simulink model "LogisticsMissionPlanEval"  (R2026a)
settings: Solver=VariableStepAuto  StopTime=CAMPAIGN_HR
undefined symbols (not defined in the file or in its folder): DISPATCH_PERIOD_HR, DORMANT_FACTOR, FOB_CONSUMPTION_TPH, FOB_STOCK_INITIAL_TONS, LOSS_FRAC_MAX, LOSS_FRAC_MIN, m, n, P_AMBUSH_NORTH, P_AMBUSH_SOUTH, P_CATASTROPHIC_KILL, RUN_SEED_NORTH, RUN_SEED_SOUTH, SURGE_FACTOR, T_ACTIVE_NORTH_HR, T_ACTIVE_SOUTH_HR, T_DORMANT_NORTH_HR, T_DORMANT_SOUTH_HR, T_SURGE_NORTH_HR, T_SURGE_SOUTH_HR
settings Model: Creator=sarah  LastModifiedBy=sdagen

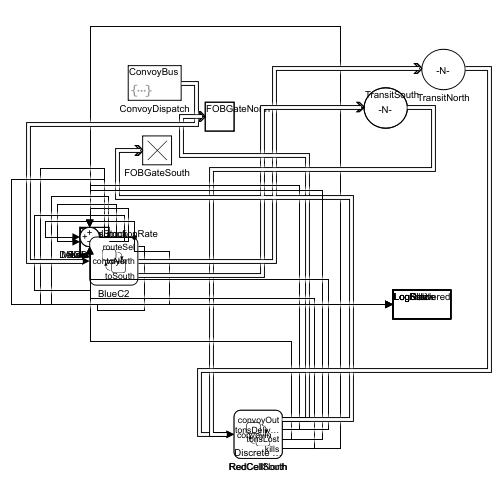
[thumbnail: Simulink's stored preview of the top-level diagram]
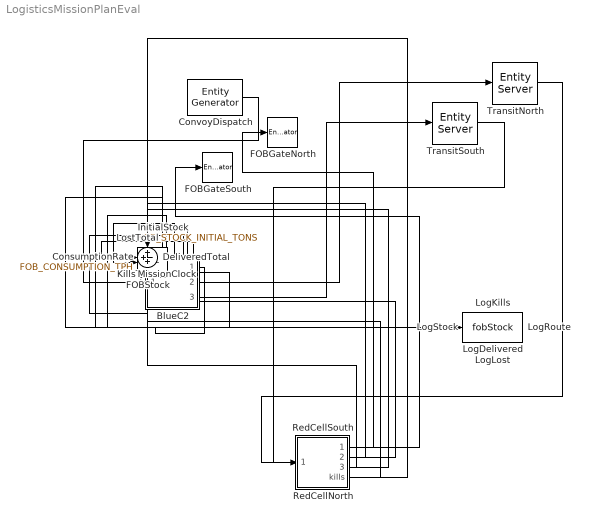
== system LogisticsMissionPlanEval ==
  BlueC2 : Stateflow chart  TreatAsAtomicUnit=on
  ConsumptionRate : Gain  Gain=FOB_CONSUMPTION_TPH
  ConvoyDispatch : EntityGenerator  OutputPortMessageModes=m  Period=DISPATCH_PERIOD_HR  GenerateAction=|  EntityType=Bus object  EntityTypeName=ConvoyBus  DataInitialValue=CONVOY_INIT
      | entity.Trucks = TRUCKS_PER_CONVOY;
      | entity.CargoTons = CONVOY_CARGO_TONS;
  DeliveredTotal : Sum
  FOBGateNorth : EntityTerminator  InputPortMessageModes=m
  FOBGateSouth : EntityTerminator  InputPortMessageModes=m
  FOBStock : Sum  Inputs=++-
  InitialStock : Constant  Value=FOB_STOCK_INITIAL_TONS
  KillsTotal : Sum
  LogDelivered : ToWorkspace  VariableName=deliveredTons  SaveFormat=Timeseries  SampleTime=-1
  LogKills : ToWorkspace  VariableName=convoysKilled  SaveFormat=Timeseries  SampleTime=-1
  LogLost : ToWorkspace  VariableName=lostTons  SaveFormat=Timeseries  SampleTime=-1
  LogRoute : ToWorkspace  VariableName=routeSelected  SaveFormat=Timeseries  SampleTime=-1
  LogStock : ToWorkspace  VariableName=fobStock  SaveFormat=Timeseries  SampleTime=-1
  LostTotal : Sum
  MissionClock : Clock
  RedCellNorth : Stateflow chart  TreatAsAtomicUnit=on
  RedCellSouth : Stateflow chart  TreatAsAtomicUnit=on
  TransitNorth : EntityServer  InputPortMessageModes=m  OutputPortMessageModes=m  Capacity=MAX_CONVOYS_EN_ROUTE  ServiceTimeValue=TRANSIT_NORTH_HR
  TransitSouth : EntityServer  InputPortMessageModes=m  OutputPortMessageModes=m  Capacity=MAX_CONVOYS_EN_ROUTE  ServiceTimeValue=TRANSIT_SOUTH_HR
  wires:
  MissionClock/1 -> ConsumptionRate/1
  InitialStock/1 -> FOBStock/1
  DeliveredTotal/1 -> LogDelivered/1, FOBStock/2
  ConsumptionRate/1 -> FOBStock/3
  LostTotal/1 -> LogLost/1
  KillsTotal/1 -> LogKills/1
  FOBStock/1 -> LogStock/1
  TransitNorth/1 -> RedCellNorth/1(convoyIn)
  TransitSouth/1 -> RedCellSouth/1(convoyIn)
  RedCellNorth/1(convoyOut) -> FOBGateNorth/1
  RedCellSouth/1(convoyOut) -> FOBGateSouth/1
  RedCellNorth/2(tonsDelivered) -> DeliveredTotal/1
  RedCellSouth/2(tonsDelivered) -> DeliveredTotal/2
  RedCellNorth/3(tonsLost) -> LostTotal/1
  RedCellSouth/3(tonsLost) -> LostTotal/2
  RedCellNorth/4(kills) -> KillsTotal/1
  RedCellSouth/4(kills) -> KillsTotal/2
  BlueC2/1(routeSel) -> LogRoute/1
  ConvoyDispatch/1 -> BlueC2/1(convoyIn)
  BlueC2/2(toNorth) -> TransitNorth/1
  BlueC2/3(toSouth) -> TransitSouth/1

== stateflow chart LogisticsMissionPlanEval/RedCellSouth ==
  settings: enableNonTerminalStates=1
  state Posture [parallel]
    settings: executionOrder=2
    state Dormant
      en: pCur = P_AMBUSH_SOUTH * DORMANT_FACTOR;
    state Active
      en: pCur = P_AMBUSH_SOUTH;
    state Surge
      en: pCur = min(0.95, P_AMBUSH_SOUTH * SURGE_FACTOR);
    (default) -> Dormant
    Dormant -> Active : after(T_DORMANT_SOUTH_HR, sec)
    Surge -> Dormant : after(T_SURGE_SOUTH_HR, sec)
    Active -> Surge : after(T_ACTIVE_SOUTH_HR, sec)
  state Handler [parallel]
    en: rngState = max(1, mod(round(RUN_SEED_SOUTH), 2147483646));
    on convoyIn:
    if nextRand() < pCur
    if nextRand() < P_CATASTROPHIC_KILL
    tonsLost = tonsLost + convoyIn.data.CargoTons;
    kills = kills + 1;
    else
    lossFrac = LOSS_FRAC_MIN + (LOSS_FRAC_MAX - LOSS_FRAC_MIN)*nextRand();
    lostTrucks = ceil(lossFrac*convoyIn.data.Trucks);
    lostTons = lostTrucks*(convoyIn.data.CargoTons/convoyIn.data.Trucks);
    convoyIn.data.Trucks = convoyIn.data.Trucks - lostTrucks;
    convoyIn.data.CargoTons = convoyIn.data.CargoTons - lostTons;
    tonsLost = tonsLost + lostTons;
    tonsDelivered = tonsDelivered + convoyIn.data.CargoTons;
    forward(convoyIn, convoyOut);
    end
    else
    tonsDelivered = tonsDelivered + convoyIn.data.CargoTons;
    forward(convoyIn, convoyOut);
    end
    settings: executionOrder=1
  data: r function_output; convoyIn input; convoyOut output Bus: ConvoyBus; tonsDelivered output double =0; tonsLost output double =0; kills output double =0; pCur local double =0; lossFrac local double =0; lostTrucks local double =0; lostTons local double =0; P_AMBUSH_SOUTH parameter; DORMANT_FACTOR parameter; SURGE_FACTOR parameter; LOSS_FRAC_MIN parameter; LOSS_FRAC_MAX parameter; P_CATASTROPHIC_KILL parameter; T_DORMANT_SOUTH_HR parameter; T_ACTIVE_SOUTH_HR parameter; T_SURGE_SOUTH_HR parameter; RUN_SEED_SOUTH parameter; rngState local double =1
  function r = nextRand:
    | function r = nextRand
    | % Park-Miller minimal standard LCG on chart-local state.
    | % Keeps campaign realizations reproducible per RUN_SEED value.
    | rngState = mod(16807 * rngState, 2147483647);
    | if rngState == 0
    |     rngState = 1;
    | end
    | r = rngState / 2147483647;
    | end

== stateflow chart LogisticsMissionPlanEval/BlueC2 ==
  state Assess
    on convoyIn:
    routeSel = round(ROUTE_PLAN_SEQUENCE(min(planIdx, numel(ROUTE_PLAN_SEQUENCE))));
    routeSel = max(1, min(2, routeSel));
    if routeSel == 1
    forward(convoyIn, toNorth);
    else
    forward(convoyIn, toSouth);
    end
    planIdx = min(planIdx + 1, numel(ROUTE_PLAN_SEQUENCE));
  (default) -> Assess : {routeSel = 1; planIdx = 1;}
  data: routeSel output double =1; convoyIn input; toNorth output Bus: ConvoyBus; toSouth output Bus: ConvoyBus; planIdx local double; ROUTE_PLAN_SEQUENCE parameter double

== stateflow chart LogisticsMissionPlanEval/RedCellNorth ==
  settings: enableNonTerminalStates=1
  state Posture [parallel]
    settings: executionOrder=2
    state Dormant
      en: pCur = P_AMBUSH_NORTH * DORMANT_FACTOR;
    state Active
      en: pCur = P_AMBUSH_NORTH;
    state Surge
      en: pCur = min(0.95, P_AMBUSH_NORTH * SURGE_FACTOR);
    (default) -> Dormant
    Dormant -> Active : after(T_DORMANT_NORTH_HR, sec)
    Surge -> Dormant : after(T_SURGE_NORTH_HR, sec)
    Active -> Surge : after(T_ACTIVE_NORTH_HR, sec)
  state Handler [parallel]
    en: rngState = max(1, mod(round(RUN_SEED_NORTH), 2147483646));
    on convoyIn:
    if nextRand() < pCur
    if nextRand() < P_CATASTROPHIC_KILL
    tonsLost = tonsLost + convoyIn.data.CargoTons;
    kills = kills + 1;
    else
    lossFrac = LOSS_FRAC_MIN + (LOSS_FRAC_MAX - LOSS_FRAC_MIN)*nextRand();
    lostTrucks = ceil(lossFrac*convoyIn.data.Trucks);
    lostTons = lostTrucks*(convoyIn.data.CargoTons/convoyIn.data.Trucks);
    convoyIn.data.Trucks = convoyIn.data.Trucks - lostTrucks;
    convoyIn.data.CargoTons = convoyIn.data.CargoTons - lostTons;
    tonsLost = tonsLost + lostTons;
    tonsDelivered = tonsDelivered + convoyIn.data.CargoTons;
    forward(convoyIn, convoyOut);
    end
    else
    tonsDelivered = tonsDelivered + convoyIn.data.CargoTons;
    forward(convoyIn, convoyOut);
    end
    settings: executionOrder=1
  data: r function_output; convoyIn input; convoyOut output Bus: ConvoyBus; tonsDelivered output double =0; tonsLost output double =0; kills output double =0; pCur local double =0; lossFrac local double =0; lostTrucks local double =0; lostTons local double =0; P_AMBUSH_NORTH parameter; DORMANT_FACTOR parameter; SURGE_FACTOR parameter; LOSS_FRAC_MIN parameter; LOSS_FRAC_MAX parameter; P_CATASTROPHIC_KILL parameter; T_DORMANT_NORTH_HR parameter; T_ACTIVE_NORTH_HR parameter; T_SURGE_NORTH_HR parameter; RUN_SEED_NORTH parameter; rngState local double =1
  function r = nextRand:
    | function r = nextRand
    | % Park-Miller minimal standard LCG on chart-local state.
    | % Keeps campaign realizations reproducible per RUN_SEED value.
    | rngState = mod(16807 * rngState, 2147483647);
    | if rngState == 0
    |     rngState = 1;
    | end
    | r = rngState / 2147483647;
    | end
